simulink model "c_station_v2"  (R2019a)
settings: Solver=VariableStepAuto  StartTime=0.0  StopTime=604800  MaxStep=3600  RelTol=1e-3  AbsTol=1e-3  EnableMultiTasking=on
values from neighbouring files (symbols this model uses):
  conf = gasConfig()    [gas_v1.m]
  loadControlFlag = "on"    [gas_v1.m]
  valveControlFlag = "on"    [gas_v1.m]
undefined symbols (not defined in the file or in its folder): f, lineParm, loadParm, valveParm
libraries: fl_lib x31, gasLibrary x13, nesl_utility x13, instrumentlib x6, SimscapeFluids_lib x1
(part 3 of 3)

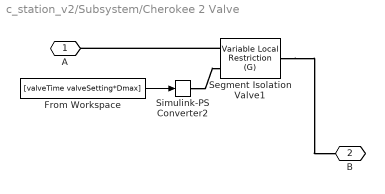
== system c_station_v2/Subsystem/Cherokee 2 Valve ==
  From Workspace : FromWorkspace  VariableName=[valveTime valveSetting*Dmax]  SampleTime=0  OutputAfterFinalValue=Holding final value
  Segment Isolation Valve1 : fl_lib/Gas/Elements/Variable Local Restriction (G)  min_area=1e-4 in^2  max_area=pi*(Dmax-1)^2/4 in^2  area=pi*D^2/4 in^2  Cd=0.64  B_lam=0.999  mdot_A_specify=off  mdot_A_priority=None  mdot_A=1e-6 kg/s  mdot_A_nominal_specify=off  mdot_A_nominal_unit=kg/s  mdot_A_nominal_value=1
      settings: SourceProductName=Simscape  SourceProductBaseCode=SS
  Simulink-PS Converter2 : nesl_utility/Simulink-PS Converter  PhysicalDomain=network_engine_domain  SubClassName=ps_input  LeftPortType=input  RightPortType=output  PseudoPeriodic=off  Frequencies=[]  NoiseDistribution=none  NoiseParameters=[]  Unit=in^2  AffineConversion=off  FilteringAndDerivatives=provide  SimscapeFilterOrder=1  InputFilterTimeConstant=0.001  UdotUserProvided=0
  A : PMIOPort  Side=Left
  B : PMIOPort  Port=2  Side=Right
  wires:
  From Workspace/1 -> Simulink-PS Converter2/1
  connections:
  Simulink-PS Converter2/RConn1 -- Segment Isolation Valve1/LConn2
  Segment Isolation Valve1/LConn1 -- A/RConn1
  Segment Isolation Valve1/RConn1 -- B/RConn1

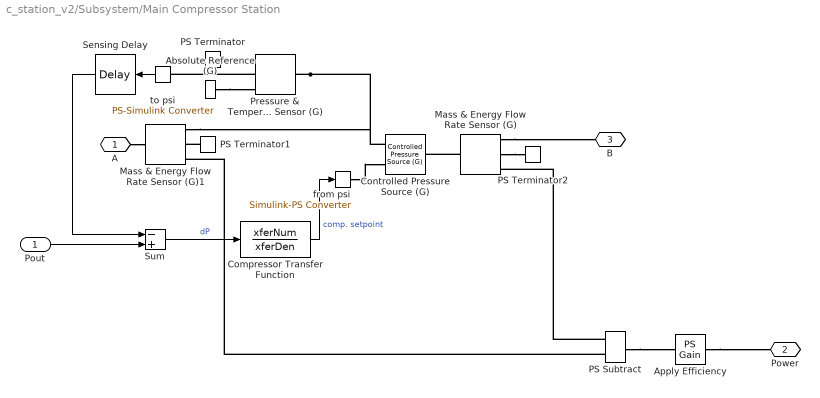
== system c_station_v2/Subsystem/Main Compressor Station ==
  Pout : Inport
  Absolute Reference (G) : fl_lib/Gas/Elements/Absolute Reference (G)
      settings: SourceProductName=Simscape  SourceProductBaseCode=SS
  Apply Efficiency : fl_lib/Physical Signals/Functions/PS Gain  gain=1/efficiency
  Compressor Transfer Function : TransferFcn  Numerator=xferNum  Denominator=xferDen
  Controlled Pressure Source (G) : fl_lib/Gas/Sources/Controlled Pressure Source (G)  power_spec=1  area_A=24^2*pi/4 in^2  area_B=24^2*pi/4 in^2  mdot_A_specify=off  mdot_A_priority=None  mdot_A=1e-6 kg/s  mdot_A_nominal_specify=off  mdot_A_nominal_unit=kg/s  mdot_A_nominal_value=1
      settings: SourceProductName=Simscape  SourceProductBaseCode=SS
  Mass & Energy Flow Rate Sensor (G) : fl_lib/Gas/Sensors/Mass & Energy Flow Rate Sensor (G)
      settings: SourceProductName=Simscape  SourceProductBaseCode=SS
  Mass & Energy Flow Rate Sensor (G)1 : fl_lib/Gas/Sensors/Mass & Energy Flow Rate Sensor (G)
      settings: SourceProductName=Simscape  SourceProductBaseCode=SS
  PS Subtract : fl_lib/Physical Signals/Functions/PS Subtract
      settings: SourceProductName=Simscape
  PS Terminator : fl_lib/Physical Signals/Sinks/PS Terminator
      settings: SourceProductName=Simscape
  PS Terminator1 : fl_lib/Physical Signals/Sinks/PS Terminator
      settings: SourceProductName=Simscape
  PS Terminator2 : fl_lib/Physical Signals/Sinks/PS Terminator
      settings: SourceProductName=Simscape
  Pressure & Temperature Sensor (G) : fl_lib/Gas/Sensors/Pressure & Temperature Sensor (G)
      settings: SourceProductName=Simscape  SourceProductBaseCode=SS
  Sensing Delay : TransportDelay  DelayTime=delaySeconds  TransDelayFeedthrough=on
  Sum : Sum  Inputs=-+
  from psi : nesl_utility/Simulink-PS Converter  PhysicalDomain=network_engine_domain  SubClassName=ps_input  LeftPortType=input  RightPortType=output  PseudoPeriodic=off  Frequencies=[]  NoiseDistribution=none  NoiseParameters=[]  Unit=psi  AffineConversion=off  FilteringAndDerivatives=provide  SimscapeFilterOrder=1  InputFilterTimeConstant=0.001  UdotUserProvided=0
  to psi : nesl_utility/PS-Simulink Converter  PhysicalDomain=network_engine_domain  SubClassName=ps_output  LeftPortType=input  RightPortType=output  PseudoPeriodic=off  Frequencies=[]  Unit=psi  AffineConversion=off
  A : PMIOPort  Side=Left
  Power : PMIOPort  Port=2  Side=Right
  B : PMIOPort  Port=3  Side=Right
  wires:
  to psi/1 -> Sensing Delay/1
  Sensing Delay/1 -> Sum/1
  Compressor Transfer Function/1 -> from psi/1  "comp. setpoint"
  Sum/1 -> Compressor Transfer Function/1  "dP"
  Pout/1 -> Sum/2
  connections:
  Apply Efficiency/RConn1 -- Power/RConn1
  PS Subtract/RConn1 -- Apply Efficiency/LConn1
  PS Subtract/LConn2 -- Mass & Energy Flow Rate Sensor (G)1/RConn3
  PS Subtract/LConn1 -- Mass & Energy Flow Rate Sensor (G)/RConn3
  Mass & Energy Flow Rate Sensor (G)/RConn2 -- PS Terminator2/LConn1
  PS Terminator1/LConn1 -- Mass & Energy Flow Rate Sensor (G)1/RConn2
  A/RConn1 -- Mass & Energy Flow Rate Sensor (G)1/LConn1
  Mass & Energy Flow Rate Sensor (G)/RConn1 -- B/RConn1
  Mass & Energy Flow Rate Sensor (G)/LConn1 -- Controlled Pressure Source (G)/RConn1
  Pressure & Temperature Sensor (G)/LConn1 -- Mass & Energy Flow Rate Sensor (G)1/RConn1 -- Controlled Pressure Source (G)/LConn1
  PS Terminator/LConn1 -- Pressure & Temperature Sensor (G)/RConn3
  from psi/RConn1 -- Controlled Pressure Source (G)/LConn2
  Pressure & Temperature Sensor (G)/RConn2 -- to psi/LConn1
  Absolute Reference (G)/LConn1 -- Pressure & Temperature Sensor (G)/RConn1

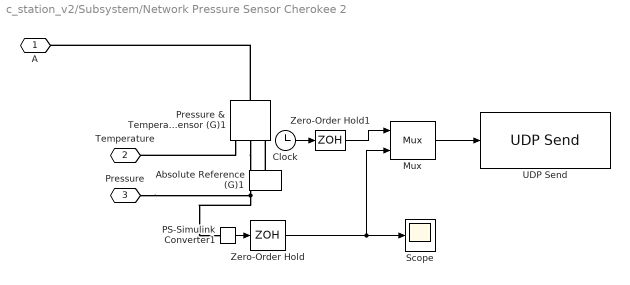
== system c_station_v2/Subsystem/Network Pressure Sensor Cherokee 2 ==
  Absolute Reference (G)1 : fl_lib/Gas/Elements/Absolute Reference (G)
      settings: SourceProductName=Simscape  SourceProductBaseCode=SS
  Clock : Clock
  Mux : Mux  Inputs=2
      settings: DisplayOption=signals
  PS-Simulink Converter1 : nesl_utility/PS-Simulink Converter  PhysicalDomain=network_engine_domain  SubClassName=ps_output  LeftPortType=input  RightPortType=output  PseudoPeriodic=off  Frequencies=[]  Unit=1  AffineConversion=off
  Pressure & Temperature Sensor (G)1 : fl_lib/Gas/Sensors/Pressure & Temperature Sensor (G)
      settings: SourceProductName=Simscape  SourceProductBaseCode=SS
  Scope : Scope
  UDP Send : instrumentlib/UDP Send  Host=localhost  Port=7070  LocalPort=-1  EnablePortSharing=off  ByteOrder=BigEndian  OutputDatagramPacketSize=512  EnableBlockingMode=off  LocalAddress=0.0.0.0
      settings: SourceProductName=Instrument Control Toolbox
  Zero-Order Hold : ZeroOrderHold  SampleTime=300
  Zero-Order Hold1 : ZeroOrderHold  SampleTime=-1
  A : PMIOPort  Side=Left
  Temperature : PMIOPort  Port=2  Side=Right
  Pressure : PMIOPort  Port=3  Side=Right
  wires:
  PS-Simulink Converter1/1 -> Zero-Order Hold/1
  Zero-Order Hold/1 -> Scope/1, Mux/2
  Mux/1 -> UDP Send/1
  Clock/1 -> Zero-Order Hold1/1
  Zero-Order Hold1/1 -> Mux/1
  connections:
  Absolute Reference (G)1/LConn1 -- Pressure & Temperature Sensor (G)1/RConn1
  Pressure & Temperature Sensor (G)1/RConn2 -- PS-Simulink Converter1/LConn1 -- Pressure/RConn1
  Pressure & Temperature Sensor (G)1/LConn1 -- A/RConn1
  Pressure & Temperature Sensor (G)1/RConn3 -- Temperature/RConn1

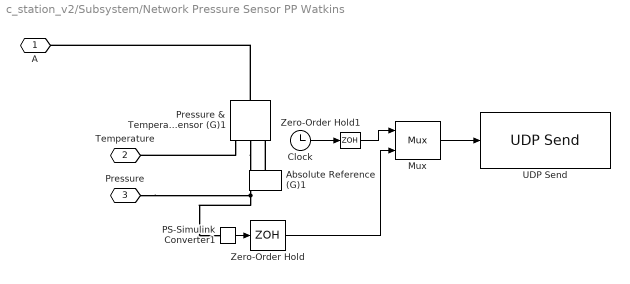
== system c_station_v2/Subsystem/Network Pressure Sensor PP Watkins ==
  Absolute Reference (G)1 : fl_lib/Gas/Elements/Absolute Reference (G)
      settings: SourceProductName=Simscape  SourceProductBaseCode=SS
  Clock : Clock
  Mux : Mux  Inputs=2
      settings: DisplayOption=signals
  PS-Simulink Converter1 : nesl_utility/PS-Simulink Converter  PhysicalDomain=network_engine_domain  SubClassName=ps_output  LeftPortType=input  RightPortType=output  PseudoPeriodic=off  Frequencies=[]  Unit=1  AffineConversion=off
  Pressure & Temperature Sensor (G)1 : fl_lib/Gas/Sensors/Pressure & Temperature Sensor (G)
      settings: SourceProductName=Simscape  SourceProductBaseCode=SS
  UDP Send : instrumentlib/UDP Send  Host=localhost  Port=7071  LocalPort=-1  EnablePortSharing=off  ByteOrder=BigEndian  OutputDatagramPacketSize=512  EnableBlockingMode=off  LocalAddress=0.0.0.0
      settings: SourceProductName=Instrument Control Toolbox
  Zero-Order Hold : ZeroOrderHold  SampleTime=300
  Zero-Order Hold1 : ZeroOrderHold  SampleTime=-1
  A : PMIOPort  Side=Left
  Temperature : PMIOPort  Port=2  Side=Right
  Pressure : PMIOPort  Port=3  Side=Right
  wires:
  PS-Simulink Converter1/1 -> Zero-Order Hold/1
  Zero-Order Hold/1 -> Mux/2
  Mux/1 -> UDP Send/1
  Zero-Order Hold1/1 -> Mux/1
  Clock/1 -> Zero-Order Hold1/1
  connections:
  Absolute Reference (G)1/LConn1 -- Pressure & Temperature Sensor (G)1/RConn1
  Pressure & Temperature Sensor (G)1/RConn2 -- PS-Simulink Converter1/LConn1 -- Pressure/RConn1
  Pressure & Temperature Sensor (G)1/LConn1 -- A/RConn1
  Pressure & Temperature Sensor (G)1/RConn3 -- Temperature/RConn1

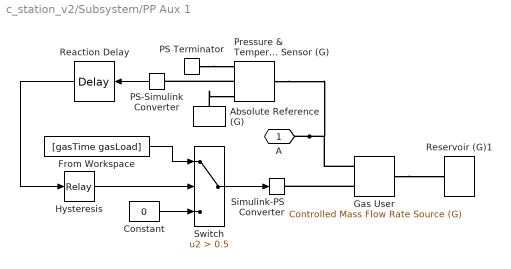
== system c_station_v2/Subsystem/PP Aux 1 ==
  Absolute Reference (G) : fl_lib/Gas/Elements/Absolute Reference (G)
      settings: SourceProductName=Simscape  SourceProductBaseCode=SS
  Constant : Constant  Value=0
  From Workspace : FromWorkspace  VariableName=[gasTime gasLoad]  SampleTime=0  OutputAfterFinalValue=Holding final value
  Gas User : fl_lib/Gas/Sources/Controlled Mass Flow Rate Source (G)  power_spec=1  area_A=24^2*pi/4 in^2  area_B=20^2*pi/4 in^2  mdot_A_specify=on  mdot_A_priority=None  mdot_A=20 kg/s  mdot_A_nominal_specify=off  mdot_A_nominal_unit=kg/s  mdot_A_nominal_value=1
      settings: SourceProductName=Simscape  SourceProductBaseCode=SS
  Hysteresis : Relay  OnSwitchValue=pCutoff*1.05  OffSwitchValue=pCutoff
  PS Terminator : fl_lib/Physical Signals/Sinks/PS Terminator
      settings: SourceProductName=Simscape
  PS-Simulink Converter : nesl_utility/PS-Simulink Converter  PhysicalDomain=network_engine_domain  SubClassName=ps_output  LeftPortType=input  RightPortType=output  PseudoPeriodic=off  Frequencies=[]  Unit=psi  AffineConversion=off
  Pressure & Temperature Sensor (G) : fl_lib/Gas/Sensors/Pressure & Temperature Sensor (G)
      settings: SourceProductName=Simscape  SourceProductBaseCode=SS
  Reaction Delay : TransportDelay  DelayTime=60  InitialOutput=pNominal
  Reservoir (G)1 : fl_lib/Gas/Elements/Reservoir (G)  pressure_spec=2  reservoir_pressure=300 psi  reservoir_temperature=25 degC  area_A=pi*25^2/4 in^2
      settings: SourceProductName=Foundation Library
  Simulink-PS Converter : nesl_utility/Simulink-PS Converter  PhysicalDomain=network_engine_domain  SubClassName=ps_input  LeftPortType=input  RightPortType=output  PseudoPeriodic=off  Frequencies=[]  NoiseDistribution=none  NoiseParameters=[]  Unit=1  AffineConversion=off  FilteringAndDerivatives=provide  SimscapeFilterOrder=1  InputFilterTimeConstant=0.001  UdotUserProvided=0
  Switch : Switch  Criteria=u2 > Threshold  Threshold=0.5
  A : PMIOPort  Side=Left
  wires:
  Hysteresis/1 -> Switch/2
  Constant/1 -> Switch/3
  From Workspace/1 -> Switch/1
  PS-Simulink Converter/1 -> Reaction Delay/1
  Reaction Delay/1 -> Hysteresis/1
  Switch/1 -> Simulink-PS Converter/1
  connections:
  Pressure & Temperature Sensor (G)/RConn2 -- PS-Simulink Converter/LConn1
  Absolute Reference (G)/LConn1 -- Pressure & Temperature Sensor (G)/RConn1
  PS Terminator/LConn1 -- Pressure & Temperature Sensor (G)/RConn3
  Gas User/LConn2 -- Simulink-PS Converter/RConn1
  A/RConn1 -- Pressure & Temperature Sensor (G)/LConn1 -- Gas User/LConn1
  Gas User/RConn1 -- Reservoir (G)1/LConn1

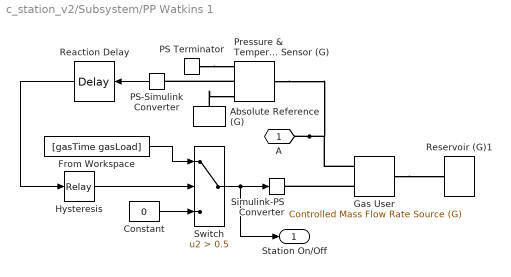
== system c_station_v2/Subsystem/PP Watkins 1 ==
  Absolute Reference (G) : fl_lib/Gas/Elements/Absolute Reference (G)
      settings: SourceProductName=Simscape  SourceProductBaseCode=SS
  Constant : Constant  Value=0
  From Workspace : FromWorkspace  VariableName=[gasTime gasLoad]  SampleTime=0  OutputAfterFinalValue=Holding final value
  Gas User : fl_lib/Gas/Sources/Controlled Mass Flow Rate Source (G)  power_spec=1  area_A=24^2*pi/4 in^2  area_B=20^2*pi/4 in^2  mdot_A_specify=on  mdot_A_priority=None  mdot_A=20 kg/s  mdot_A_nominal_specify=off  mdot_A_nominal_unit=kg/s  mdot_A_nominal_value=1
      settings: SourceProductName=Simscape  SourceProductBaseCode=SS
  Hysteresis : Relay  OnSwitchValue=pCutoff*1.05  OffSwitchValue=pCutoff
  PS Terminator : fl_lib/Physical Signals/Sinks/PS Terminator
      settings: SourceProductName=Simscape
  PS-Simulink Converter : nesl_utility/PS-Simulink Converter  PhysicalDomain=network_engine_domain  SubClassName=ps_output  LeftPortType=input  RightPortType=output  PseudoPeriodic=off  Frequencies=[]  Unit=psi  AffineConversion=off
  Pressure & Temperature Sensor (G) : fl_lib/Gas/Sensors/Pressure & Temperature Sensor (G)
      settings: SourceProductName=Simscape  SourceProductBaseCode=SS
  Reaction Delay : TransportDelay  DelayTime=60  InitialOutput=pNominal
  Reservoir (G)1 : fl_lib/Gas/Elements/Reservoir (G)  pressure_spec=2  reservoir_pressure=300 psi  reservoir_temperature=25 degC  area_A=pi*25^2/4 in^2
      settings: SourceProductName=Foundation Library
  Simulink-PS Converter : nesl_utility/Simulink-PS Converter  PhysicalDomain=network_engine_domain  SubClassName=ps_input  LeftPortType=input  RightPortType=output  PseudoPeriodic=off  Frequencies=[]  NoiseDistribution=none  NoiseParameters=[]  Unit=1  AffineConversion=off  FilteringAndDerivatives=provide  SimscapeFilterOrder=1  InputFilterTimeConstant=0.001  UdotUserProvided=0
  Switch : Switch  Criteria=u2 > Threshold  Threshold=0.5
  A : PMIOPort  Side=Left
  "Station On/Off " : Outport
  wires:
  Hysteresis/1 -> Switch/2
  Constant/1 -> Switch/3
  From Workspace/1 -> Switch/1
  PS-Simulink Converter/1 -> Reaction Delay/1
  Reaction Delay/1 -> Hysteresis/1
  Switch/1 -> "Station On/Off "/1, Simulink-PS Converter/1
  connections:
  Pressure & Temperature Sensor (G)/RConn2 -- PS-Simulink Converter/LConn1
  Absolute Reference (G)/LConn1 -- Pressure & Temperature Sensor (G)/RConn1
  PS Terminator/LConn1 -- Pressure & Temperature Sensor (G)/RConn3
  Gas User/LConn2 -- Simulink-PS Converter/RConn1
  A/RConn1 -- Pressure & Temperature Sensor (G)/LConn1 -- Gas User/LConn1
  Gas User/RConn1 -- Reservoir (G)1/LConn1

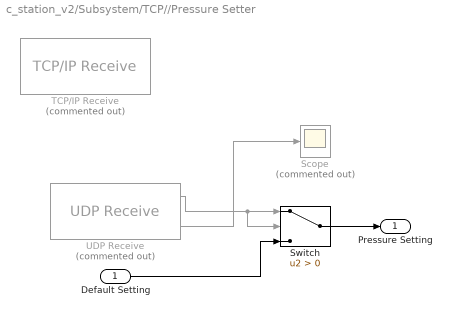
== system c_station_v2/Subsystem/TCP//Pressure Setter ==
  Default Setting : Inport
  Scope : Scope  Commented=on
  Switch : Switch  Criteria=u2 > Threshold
  TCP/IP Receive : instrumentlib/TCP//IP Receive  Commented=on  Host=localhost  Port=7777  DataSize=[1 1]  EnableBlockingMode=off  Timeout=10  SampleTime=300  DataType=int16  ByteOrder=BigEndian  ASCIIFormatting=%f,  Terminator=LF
      settings: SourceProductName=Instrument Control Toolbox
  UDP Receive : instrumentlib/UDP Receive  Commented=on  Host=localhost  Port=9090  LocalPort=7777  EnablePortSharing=off  GetLatestData=on  DataSize=[1 1]  DataType=int16  ASCIIFormatting=%f,  Terminator=LF  ByteOrder=BigEndian  EnableBlockingMode=off  Timeout=10  SampleTime=300  LocalAddress=localhost
      settings: SourceProductName=Instrument Control Toolbox
  "Pressure Setting " : Outport
  wires:
  Default Setting/1 -> Switch/3
  Switch/1 -> "Pressure Setting "/1
  UDP Receive/1 -> Switch/2, Switch/1
  UDP Receive/2 -> Scope/1

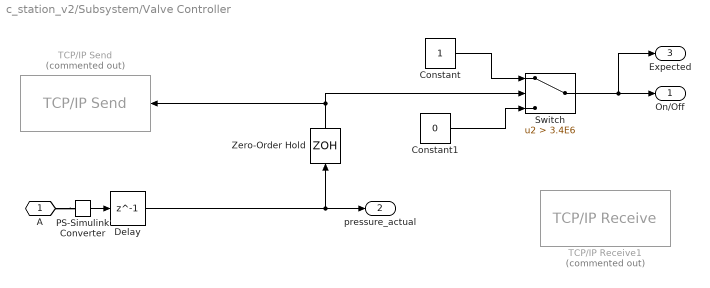
== system c_station_v2/Subsystem/Valve Controller ==
  Constant : Constant
  Constant1 : Constant  Value=0
  Delay : Delay  DelayLength=1
  PS-Simulink Converter : nesl_utility/PS-Simulink Converter  PhysicalDomain=network_engine_domain  SubClassName=ps_output  LeftPortType=input  RightPortType=output  PseudoPeriodic=off  Frequencies=[]  Unit=Pa  AffineConversion=off
  Switch : Switch  Criteria=u2 > Threshold  Threshold=3.4E6
  TCP/IP Receive1 : instrumentlib/TCP//IP Receive  Priority=2  Commented=on  Host=localhost  Port=8080  DataSize=[1 1]  EnableBlockingMode=on  Timeout=10  SampleTime=360  DataType=double  ByteOrder=BigEndian  ASCIIFormatting=%f,  Terminator=LF
      settings: SourceProductName=Instrument Control Toolbox
  TCP/IP Send : instrumentlib/TCP//IP Send  Priority=1  Commented=on  Host=localhost  Port=8080  EnableBlockingMode=on  Timeout=10  ByteOrder=BigEndian  TransferDelay=on
      settings: SourceProductName=Instrument Control Toolbox
  Zero-Order Hold : ZeroOrderHold  SampleTime=360
  A : PMIOPort  Side=Left
  On/Off : Outport
  pressure_actual : Outport  Port=2
  Expected : Outport  Port=3
  wires:
  Constant1/1 -> Switch/3
  Constant/1 -> Switch/1
  PS-Simulink Converter/1 -> Delay/1
  Delay/1 -> Zero-Order Hold/1, pressure_actual/1
  Zero-Order Hold/1 -> Switch/2, TCP/IP Send/1
  Switch/1 -> On/Off/1, Expected/1
  connections:
  A/RConn1 -- PS-Simulink Converter/LConn1

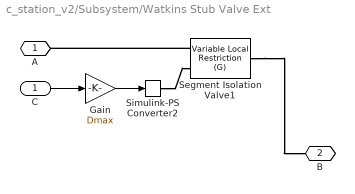
== system c_station_v2/Subsystem/Watkins Stub Valve Ext ==
  C : Inport
  Gain : Gain  Gain=Dmax
  Segment Isolation Valve1 : fl_lib/Gas/Elements/Variable Local Restriction (G)  min_area=1e-4 in^2  max_area=pi*(Dmax-1)^2/4 in^2  area=pi*D^2/4 in^2  Cd=0.64  B_lam=0.999  mdot_A_specify=off  mdot_A_priority=None  mdot_A=1e-6 kg/s  mdot_A_nominal_specify=off  mdot_A_nominal_unit=kg/s  mdot_A_nominal_value=1
      settings: SourceProductName=Simscape  SourceProductBaseCode=SS
  Simulink-PS Converter2 : nesl_utility/Simulink-PS Converter  PhysicalDomain=network_engine_domain  SubClassName=ps_input  LeftPortType=input  RightPortType=output  PseudoPeriodic=off  Frequencies=[]  NoiseDistribution=none  NoiseParameters=[]  Unit=in^2  AffineConversion=off  FilteringAndDerivatives=provide  SimscapeFilterOrder=1  InputFilterTimeConstant=0.001  UdotUserProvided=0
  A : PMIOPort  Side=Left
  B : PMIOPort  Port=2  Side=Right
  wires:
  C/1 -> Gain/1
  Gain/1 -> Simulink-PS Converter2/1
  connections:
  Segment Isolation Valve1/RConn1 -- B/RConn1
  Segment Isolation Valve1/LConn1 -- A/RConn1
  Simulink-PS Converter2/RConn1 -- Segment Isolation Valve1/LConn2
